simulink subsystem "QuadPlant"  (R2025a)
settings: Solver=VariableStepAuto  StartTime=0.0  StopTime=10.0  RelTol=1e-3
undefined symbols (not defined in the file or in its folder): cmd2thrust, cmd2torque, d, g, J, m, pos_i, Tc_m, Td_m
libraries: aerolibutil x5, matrix_library x1
settings Model: Creator=luker  LastModifiedBy=luke

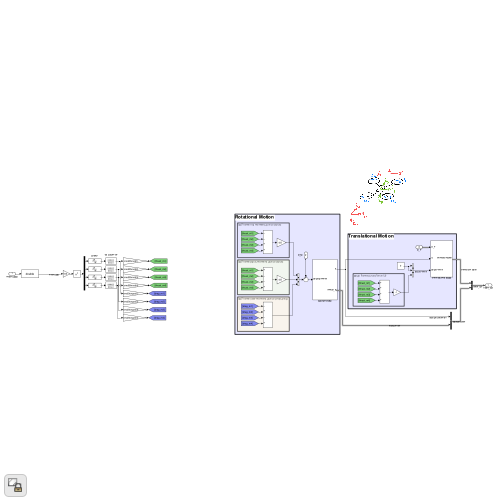
[thumbnail: Simulink's stored preview of the top-level diagram]
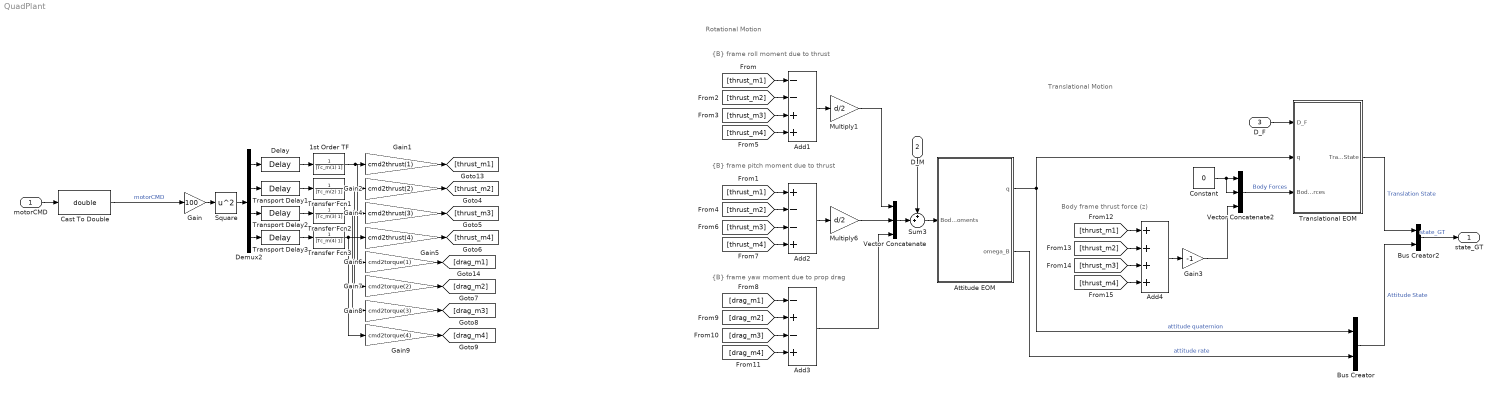
== system QuadPlant ==
  note: Translational Motion
  note: Body frame thrust force (z)
  note: {B} frame roll moment due to thrust
  note: {B} frame pitch moment due to thrust
  note: {B} frame yaw moment due to prop drag
  note: Rotational Motion
  motorCMD : Inport
  D_M : Inport  Port=2
  D_F : Inport  Port=3
  1st Order TF : TransferFcn  Denominator=[Tc_m(1) 1]
  Add1 : Sum  Inputs=--++
  Add2 : Sum  Inputs=+--+
  Add3 : Sum  Inputs=-+-+
  Add4 : Sum  Inputs=++++
  Attitude EOM : Subsystem
  Bus Creator : BusCreator  Inputs=2
  Bus Creator2 : BusCreator  Inputs=2
  Cast To Double : DataTypeConversion  OutDataTypeStr=double  SaturateOnIntegerOverflow=off  RndMeth=Floor
  Constant : Constant  Value=0
  Delay : TransportDelay  DelayTime=Td_m(1)
  Demux2 : Demux
  Gain : Gain  Gain=100
  Gain1 : Gain  Gain=cmd2thrust(1)
  Gain2 : Gain  Gain=cmd2thrust(2)
  Gain3 : Gain  Gain=-1
  Gain4 : Gain  Gain=cmd2thrust(3)
  Gain5 : Gain  Gain=cmd2thrust(4)
  Gain6 : Gain  Gain=cmd2torque(1)
  Gain7 : Gain  Gain=cmd2torque(2)
  Gain8 : Gain  Gain=cmd2torque(3)
  Gain9 : Gain  Gain=cmd2torque(4)
  Multiply1 : Gain  Gain=d/2
  Multiply6 : Gain  Gain=d/2
  Square : Math  Operator=square
  Sum3 : Sum  Inputs=++|
  Transfer Fcn1 : TransferFcn  Denominator=[Tc_m(2) 1]
  Transfer Fcn2 : TransferFcn  Denominator=[Tc_m(3) 1]
  Transfer Fcn3 : TransferFcn  Denominator=[Tc_m(4) 1]
  Translational EOM : Subsystem
  Transport Delay1 : TransportDelay  DelayTime=Td_m(2)
  Transport Delay2 : TransportDelay  DelayTime=Td_m(3)
  Transport Delay3 : TransportDelay  DelayTime=Td_m(4)
  Vector Concatenate : Concatenate  NumInputs=3
  Vector Concatenate2 : Concatenate  NumInputs=3
  state_GT : Outport
  wires:
  [thrust_m1] -> Add4/1
  Constant/1 -> Vector Concatenate2/2, Vector Concatenate2/1
  Translational EOM/1(TranslationState) -> Bus Creator2/1  "Translation State"
  Attitude EOM/2(omega_B) -> Bus Creator/2  "attitude rate"
  [thrust_m2] -> Add1/2
  Bus Creator/1 -> Bus Creator2/2  "Attitude State"
  [thrust_m4] -> Add2/4
  [thrust_m2] -> Add2/2
  Bus Creator2/1 -> state_GT/1  "state_GT"
  Add4/1 -> Gain3/1
  Add1/1 -> Multiply1/1
  [drag_m2] -> Add3/2
  [thrust_m3] -> Add1/3
  [drag_m4] -> Add3/4
  [drag_m3] -> Add3/3
  [thrust_m2] -> Add4/2
  [drag_m1] -> Add3/1
  Gain3/1 -> Vector Concatenate2/3
  [thrust_m1] -> Add2/1
  Add2/1 -> Multiply6/1
  [thrust_m4] -> Add1/4
  Attitude EOM/1(q) -> Translational EOM/2(q), Bus Creator/1  "attitude quaternion"
  [thrust_m1] -> Add1/1
  Add3/1 -> Vector Concatenate/3
  [thrust_m4] -> Add4/4
  [thrust_m3] -> Add2/3
  [thrust_m3] -> Add4/3
  Demux2/1 -> Delay/1
  Multiply6/1 -> Vector Concatenate/2
  Multiply1/1 -> Vector Concatenate/1
  Vector Concatenate/1 -> Sum3/2
  Sum3/1 -> Attitude EOM/1(Body Moments)
  D_M/1 -> Sum3/1
  Vector Concatenate2/1 -> Translational EOM/3(Body Forces)  "Body Forces"
  D_F/1 -> Translational EOM/1(D_F)
  motorCMD/1 -> Cast To Double/1
  Gain/1 -> Square/1
  Cast To Double/1 -> Gain/1  "motorCMD"
  Delay/1 -> 1st Order TF/1
  Transport Delay1/1 -> Transfer Fcn1/1
  Demux2/2 -> Transport Delay1/1
  Transport Delay2/1 -> Transfer Fcn2/1
  Transport Delay3/1 -> Transfer Fcn3/1
  Demux2/4 -> Transport Delay3/1
  Demux2/3 -> Transport Delay2/1
  Square/1 -> Demux2/1
  Gain1/1 -> [thrust_m1]
  Gain2/1 -> [thrust_m2]
  Gain4/1 -> [thrust_m3]
  Gain5/1 -> [thrust_m4]
  Gain6/1 -> [drag_m1]
  Gain7/1 -> [drag_m2]
  Gain8/1 -> [drag_m3]
  Gain9/1 -> [drag_m4]
  1st Order TF/1 -> Gain1/1, Gain6/1
  Transfer Fcn1/1 -> Gain2/1, Gain7/1
  Transfer Fcn2/1 -> Gain4/1, Gain8/1
  Transfer Fcn3/1 -> Gain5/1, Gain9/1

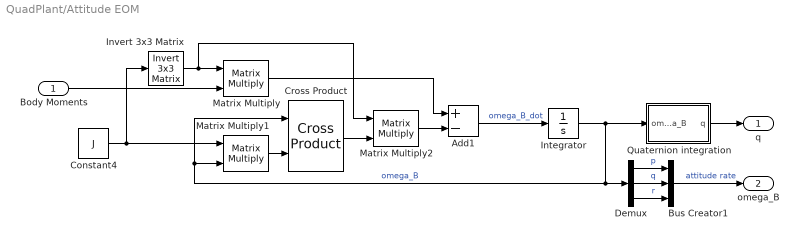
== system QuadPlant/Attitude EOM ==
  Body Moments : Inport
  Add1 : Sum  Inputs=+-
  Bus Creator1 : BusCreator  Inputs=3
  Constant4 : Constant  Value=J
  Cross Product : matrix_library/Cross Product
  Demux : Demux  Outputs=3
  Integrator : Integrator
  Invert 3x3 Matrix : aerolibutil/Invert  3x3 Matrix
  Matrix Multiply : Product  Multiplication=Matrix(*)
  Matrix Multiply1 : Product  Multiplication=Matrix(*)
  Matrix Multiply2 : Product  Multiplication=Matrix(*)
  Quaternion integration : Subsystem
  q : Outport
  omega_B : Outport  Port=2
  wires:
  Bus Creator1/1 -> omega_B/1  "attitude rate"
  Demux/3 -> Bus Creator1/3  "r"
  Demux/2 -> Bus Creator1/2  "q"
  Demux/1 -> Bus Creator1/1  "p"
  Quaternion integration/1(q) -> q/1
  Body Moments/1 -> Matrix Multiply/2
  Invert 3x3 Matrix/1 -> Matrix Multiply/1, Matrix Multiply2/1
  Integrator/1 -> Matrix Multiply1/2, Cross Product/1, Demux/1, Quaternion integration/1(omega_B)  "omega_B"
  Cross Product/1 -> Matrix Multiply2/2
  Matrix Multiply/1 -> Add1/1
  Matrix Multiply1/1 -> Cross Product/2
  Matrix Multiply2/1 -> Add1/2
  Add1/1 -> Integrator/1  "omega_B_dot"
  Constant4/1 -> Matrix Multiply1/1, Invert 3x3 Matrix/1

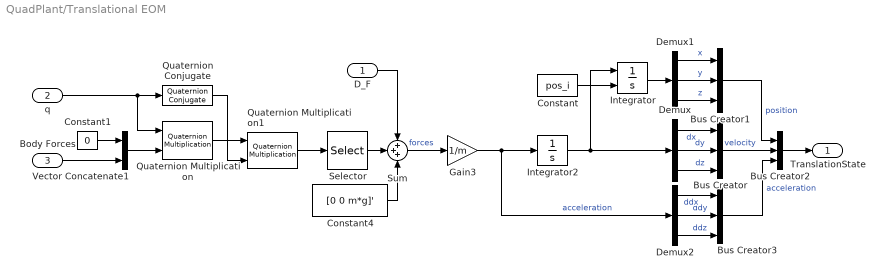
== system QuadPlant/Translational EOM ==
  D_F : Inport
  q : Inport  Port=2
  Body Forces : Inport  Port=3
  Bus Creator{,1..3} (4 alike) : BusCreator  Inputs=3
  Constant : Constant  Value=pos_i
  Constant1 : Constant  Value=0
  Constant4 : Constant  Value=[0 0 m*g]'
  Demux : Demux  Outputs=3
  Demux1 : Demux  Outputs=3
  Demux2 : Demux  Outputs=3
  Gain3 : Gain  Gain=1/m
  Integrator : Integrator  InitialConditionSource=external
  Integrator2 : Integrator
  Quaternion Conjugate : aerolibutil/Quaternion Conjugate
  Quaternion Multiplication : aerolibutil/Quaternion Multiplication
  Quaternion Multiplication1 : aerolibutil/Quaternion Multiplication
  Selector : Selector  InputPortWidth=4  IndexOptions=Index vector (dialog)  Indices=[2 3 4]  OutputSizes=1
  Sum : Sum  Inputs=+++
  Vector Concatenate1 : Concatenate
  TranslationState : Outport
  wires:
  Gain3/1 -> Integrator2/1, Demux2/1  "acceleration"
  D_F/1 -> Sum/1
  Constant4/1 -> Sum/3
  Selector/1 -> Sum/2
  Bus Creator3/1 -> Bus Creator2/3  "acceleration"
  Demux2/3 -> Bus Creator3/3  "ddz"
  Demux2/2 -> Bus Creator3/2  "ddy"
  Demux2/1 -> Bus Creator3/1  "ddx"
  Body Forces/1 -> Vector Concatenate1/2
  Integrator/1 -> Demux1/1
  Integrator2/1 -> Integrator/1, Demux/1
  Bus Creator2/1 -> TranslationState/1
  Demux1/3 -> Bus Creator1/3  "z"
  Demux1/2 -> Bus Creator1/2  "y"
  Demux1/1 -> Bus Creator1/1  "x"
  Bus Creator1/1 -> Bus Creator2/1  "position"
  Demux/3 -> Bus Creator/3  "dz"
  Demux/2 -> Bus Creator/2  "dy"
  Demux/1 -> Bus Creator/1  "dx"
  Sum/1 -> Gain3/1  "forces"
  Quaternion Multiplication1/1 -> Selector/1
  q/1 -> Quaternion Conjugate/1, Quaternion Multiplication/1
  Quaternion Multiplication/1 -> Quaternion Multiplication1/1
  Quaternion Conjugate/1 -> Quaternion Multiplication1/2
  Constant1/1 -> Vector Concatenate1/1
  Vector Concatenate1/1 -> Quaternion Multiplication/2
  Bus Creator/1 -> Bus Creator2/2  "velocity"
  Constant/1 -> Integrator/2

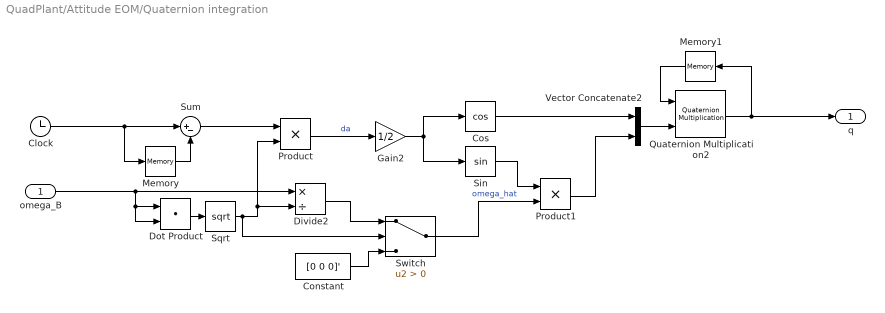
== system QuadPlant/Attitude EOM/Quaternion integration ==
  omega_B : Inport
  Clock : Clock
  Constant : Constant  Value=[0 0 0]'
  Cos : Trigonometry  Operator=cos
  Divide2 : Product  Inputs=*/
  Dot Product : DotProduct  OutDataTypeStr=Inherit: Inherit via internal rule
  Gain2 : Gain  Gain=1/2
  Memory : Memory
  Memory1 : Memory  InitialCondition=[1 0 0 0]'
  Product : Product
  Product1 : Product
  Quaternion Multiplication2 : aerolibutil/Quaternion Multiplication
  Sin : Trigonometry
  Sqrt : Sqrt
  Sum : Sum  Inputs=|+-
  Switch : Switch  Criteria=u2 > Threshold  SaturateOnIntegerOverflow=off  InputSameDT=off
  Vector Concatenate2 : Concatenate
  q : Outport
  wires:
  Dot Product/1 -> Sqrt/1
  Gain2/1 -> Cos/1, Sin/1
  Constant/1 -> Switch/3
  Vector Concatenate2/1 -> Quaternion Multiplication2/2
  Sin/1 -> Product1/1
  Clock/1 -> Memory/1, Sum/1
  Switch/1 -> Product1/2  "omega_hat"
  Cos/1 -> Vector Concatenate2/1
  Sum/1 -> Product/1
  Quaternion Multiplication2/1 -> q/1, Memory1/1
  Sqrt/1 -> Switch/2, Product/2, Divide2/2
  omega_B/1 -> Dot Product/2, Dot Product/1, Divide2/1
  Product/1 -> Gain2/1  "da"
  Memory/1 -> Sum/2
  Memory1/1 -> Quaternion Multiplication2/1
  Product1/1 -> Vector Concatenate2/2
  Divide2/1 -> Switch/1
